simulink model "TNPC_2niveis_GridConnected"  (R2023b)
settings: Solver=FixedStepDiscrete  StartTime=0.0  StopTime=0.04  RelTol=1e-3  EnableMultiTasking=on
InitFcn:
  | %% Definition of the parameters
  | 
  | Config_TNPC_Parameters
  | 
  | %% Damping
  | 
  | Rd = 4;
  | 
  | %% PRes Gains Calculation
  | 
  | % Definicao das grandezas
  | w_cl = 1j*2*pi*800;  % Phase Crossing Frequency
  | no   = 1;           % Integral Resonant Constant
  | A    = 1;             % Carrier Amplitude
  | 
  | % Kp calculation
  | a0 = 1;
  | a1 = Rd*Cf;
  | b0 = 0;
  | b1 = Lf+Lg;
  | b2 = Rd*Lf*Cf+Rd*Lg*Cf;
  | b3 = Lf*Lg*Cf;
  | 
  | G_lcl = (a1*w_cl+a0)/(b3*w_cl^3+b2*w_cl^2+b1*w_cl+b0);
  | G_lcl = 1/(Lf*w_cl+Rf);
  | 
  | G_PWM = (1/A)*(1-w_cl*Ts/4)/(1+w_cl*Ts/4);
  | 
  | G_wc  = (Vdc/2)*K_i*G_lcl*G_PWM;
  | 
  | G_wc_abs = abs(G_wc);
  | 
  | Kp = 1/G_wc_abs;
  | 
  | % Discretized Controller Gains
  | ressonance_list = [1,5];
  | 
  | n_res = length(ressonance_list);
  | a = zeros(1,n_res);
  | b = zeros(1,n_res);
  | Ki_res = zeros(1,n_res);
  | 
  | for i = 1:n_res
  |   k = ressonance_list(i);
  |   Ki_res(i) = (2.2*Kp)/(no*T_gr);
  |   a(i) = (2*Ki_res(i)*Ts)/(4+((k*w_gr)^2)*Ts^2);
  |   b(i) = (-8+2*((k*w_gr)^2)*Ts^2)/(4+((k*w_gr)^2)*Ts^2);
  | end
undefined symbols (not defined in the file): Down, GPTRIP1SEL, K_i, K_vc, K_vdc, TZ1, Up
libraries: c2802xlib x32, c2837xDlib x3, slpidlib x2
(part 2 of 2)

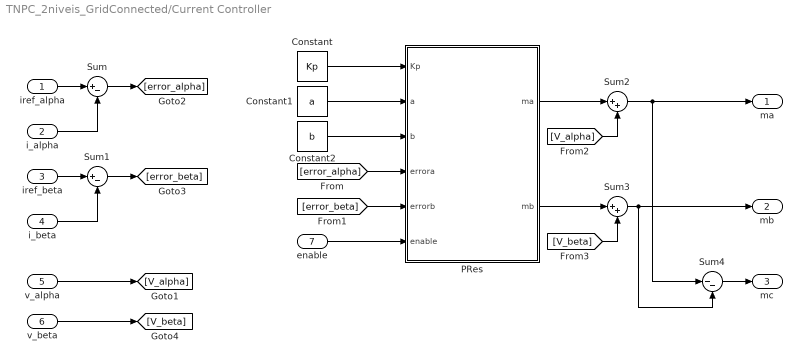
== system TNPC_2niveis_GridConnected/Current Controller ==
  iref_alpha : Inport
  i_alpha : Inport  Port=2
  iref_beta : Inport  Port=3
  i_beta : Inport  Port=4
  v_alpha : Inport  Port=5
  v_beta : Inport  Port=6
  enable : Inport  Port=7
  Constant : Constant  Value=Kp
  Constant1 : Constant  Value=a
  Constant2 : Constant  Value=b
  PRes : MATLAB Function  TreatAsAtomicUnit=on
  Sum : Sum  Inputs=|+-
  Sum1 : Sum  Inputs=|+-
  Sum2 : Sum  Inputs=|++
  Sum3 : Sum  Inputs=|++
  Sum4 : Sum  Inputs=|--
  ma : Outport
  mb : Outport  Port=2
  mc : Outport  Port=3
  wires:
  Constant/1 -> PRes/1(Kp)
  Constant1/1 -> PRes/2(a)
  Constant2/1 -> PRes/3(b)
  [error_alpha] -> PRes/4(errora)
  [error_beta] -> PRes/5(errorb)
  iref_alpha/1 -> Sum/1
  i_alpha/1 -> Sum/2
  iref_beta/1 -> Sum1/1
  i_beta/1 -> Sum1/2
  Sum1/1 -> [error_beta]
  Sum/1 -> [error_alpha]
  enable/1 -> PRes/6(enable)
  PRes/1(ma) -> Sum2/1
  Sum2/1 -> Sum4/1, ma/1
  PRes/2(mb) -> Sum3/1
  Sum3/1 -> mb/1, Sum4/2
  v_alpha/1 -> [V_alpha]
  v_beta/1 -> [V_beta]
  [V_alpha] -> Sum2/2
  [V_beta] -> Sum3/2
  Sum4/1 -> mc/1

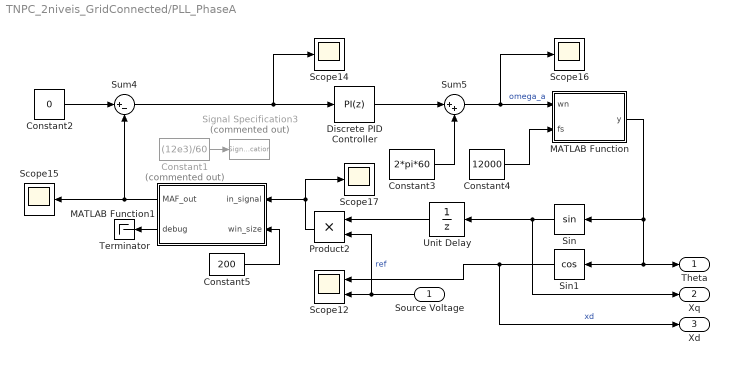
== system TNPC_2niveis_GridConnected/PLL_PhaseA ==
  Source Voltage : Inport
  Constant1 : Constant  Commented=on  Value=(12e3)/60
  Constant2 : Constant  Value=0  OutDataTypeStr=single
  Constant3 : Constant  Value=2*pi*60  OutDataTypeStr=single
  Constant4 : Constant  Value=12000  OutDataTypeStr=single
  Constant5 : Constant  Value=200  OutDataTypeStr=single
  Discrete PID Controller : slpidlib/PID Controller  Controller=PI  Form=Parallel  TimeDomain=Discrete-time  UseExternalTs=off  SampleTime=-1  IntegratorMethod=Forward Euler  FilterMethod=Forward Euler  ControllerParametersSource=internal  P=200  I=4000  UseKiTs=off  D=0  N=100  UseFilter=on  TunerSelectOption=Transfer Function Based (PID Tuner App)  InitialConditionSource=internal  InitialConditionForIntegrator=0  InitialConditionForFilter=0  DifferentiatorICPrevScaledInput=0  ExternalReset=none  TrackingMode=off  Kt=1  LimitOutput=off  SatLimitsSource=internal  UpperSaturationLimit=inf  LowerSaturationLimit=-inf  LinearizeAsGain=off  AntiWindupMode=none  Kb=1  LimitIntegrator=off  UpperIntegratorSaturationLimit=inf  LowerIntegratorSaturationLimit=-inf  POutMin=[]  POutMax=[]  IOutMin=[]  IOutMax=[]  DOutMin=[]  DOutMax=[]  NOutMin=[]  NOutMax=[]  SumOutMin=[]  SumOutMax=[]  SaturationOutMin=[]  SaturationOutMax=[]  PParamMin=[]  PParamMax=[]  IParamMin=[]  IParamMax=[]  DParamMin=[]  DParamMax=[]  NParamMin=[]  NParamMax=[]  KbParamMin=[]  KbParamMax=[]  KtParamMin=[]  KtParamMax=[]  KbOutMin=[]  KbOutMax=[]  KtOutMin=[]  KtOutMax=[]  IntegratorOutMin=[]  IntegratorOutMax=[]  FilterOutMin=[]  FilterOutMax=[]  SumI1OutMin=[]  SumI1OutMax=[]  SumI2OutMin=[]  SumI2OutMax=[]  SumI3OutMin=[]  SumI3OutMax=[]  SumI4OutMin=[]  SumI4OutMax=[]  SumDOutMin=[]  SumDOutMax=[]  DifferentiatorOutMin=[]  DifferentiatorOutMax=[]  FilterDiffOutCoefMin=[]  FilterDiffOutCoefMax=[]  ReciprocalOutMin=[]  ReciprocalOutMax=[]  SumDenOutMin=[]  SumDenOutMax=[]  SumNumOutMin=[]  SumNumOutMax=[]  DivideOutMin=[]  DivideOutMax=[]  UdiffTsProdOutMin=[]  UdiffTsProdOutMax=[]  NTsProdOutMin=[]  NTsProdOutMax=[]  UintegralTsProdOutMin=[]  UintegralTsProdOutMax=[]  UngainTsProdOutMin=[]  UngainTsProdOutMax=[]  ClampingZeroOutDataTypeStr=Inherit: Inherit via back propagation  ClampingZeroOutMin=[]  ClampingZeroOutMax=[]  FilterDenConstantOutDataTypeStr=Inherit: Inherit via back propagation  FilterDenConstantOutMin=[]  FilterDenConstantOutMax=[]  PCopyOutDataTypeStr=Inherit: Inherit via back propagation  PCopyOutMin=[]  PCopyOutMax=[]  NCopyOutDataTypeStr=Inherit: Inherit via back propagation  NCopyOutMin=[]  NCopyOutMax=[]  IntegratorContinuousStateAttributes=''  IntegratorStateMustResolveToSignalObject=off  IntegratorRTWStateStorageClass=Auto  FilterContinuousStateAttributes=''  FilterStateMustResolveToSignalObject=off  FilterRTWStateStorageClass=Auto  ParallelPVariant=InternalParameters  IdealPVariant=Disabled  IVariant=InternalParameters  DVariant=Disabled  IntegratorVariant=Discrete  SatVariant=Disabled  AWVariant=Passthrough  PCopyVariant=Disabled  TRVariant=Disabled  FdbkBlocksVariant=Forward  IdealPFdbkVariant=Disabled  SatFdbkVariant=Disabled  DerivativeFilterVariant=Disabled  NVariant=Disabled  NCopyVariant=Disabled_SignalSpec  FilterICVariant=Disabled  IntegratorICVariant=InternalICs  ExternalResetVariant=Disabled  TRSumVariant=Passthrough  SumFdbkVariant=Disabled  SumVariant=Sum_PI  TsampFilterVariant=InternalTs  TsampNgainVariant=Passthrough  TsampIntegralVariant=Disabled_SignalSpec  ExternalSaturationOutDataTypeStr=Inherit: Same as second input
  MATLAB Function : MATLAB Function  TreatAsAtomicUnit=on
  MATLAB Function1 : MATLAB Function  TreatAsAtomicUnit=on
  Product2 : Product
  Scope12 : Scope  NumInputPorts=2
  Scope{14..17} (4 alike) : Scope
  Signal Specification3 : SignalSpecification  Commented=on  Dimensions=[1 1]
  Sin : Trigonometry
  Sin1 : Trigonometry  Operator=cos
  Sum4 : Sum  Inputs=|+-
  Sum5 : Sum  Inputs=|++
  Terminator : Terminator
  Unit Delay : UnitDelay  SampleTime=-1  HasFrameUpgradeWarning=on
  Theta : Outport
  Xq : Outport  Port=2
  Xd : Outport  Port=3
  wires:
  Constant1/1 -> Signal Specification3/1
  Constant4/1 -> MATLAB Function/2(fs)
  Sum5/1 -> MATLAB Function/1(wn), Scope16/1  "omega_a"
  Source Voltage/1 -> Scope12/2, Product2/2  "ref"
  Constant3/1 -> Sum5/2
  Unit Delay/1 -> Product2/1
  Constant2/1 -> Sum4/1
  Sum4/1 -> Scope14/1, Discrete PID Controller/1
  Sin/1 -> Unit Delay/1, Xq/1
  Sin1/1 -> Scope12/1, Xd/1  "xd"
  Product2/1 -> MATLAB Function1/1(in_signal), Scope17/1
  MATLAB Function/1(y) -> Sin/1, Sin1/1, Theta/1
  Discrete PID Controller/1 -> Sum5/1
  MATLAB Function1/1(MAF_out) -> Sum4/2, Scope15/1
  Constant5/1 -> MATLAB Function1/2(win_size)
  MATLAB Function1/2(debug) -> Terminator/1

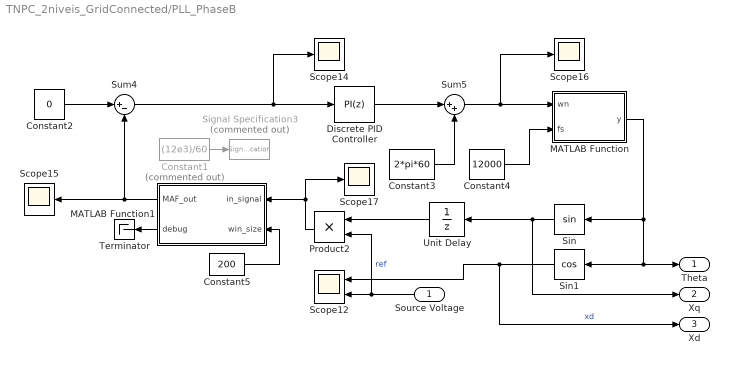
== system TNPC_2niveis_GridConnected/PLL_PhaseB ==
  Source Voltage : Inport
  Constant1 : Constant  Commented=on  Value=(12e3)/60
  Constant2 : Constant  Value=0  OutDataTypeStr=single
  Constant3 : Constant  Value=2*pi*60  OutDataTypeStr=single
  Constant4 : Constant  Value=12000  OutDataTypeStr=single
  Constant5 : Constant  Value=200  OutDataTypeStr=single
  Discrete PID Controller : slpidlib/PID Controller  Controller=PI  Form=Parallel  TimeDomain=Discrete-time  UseExternalTs=off  SampleTime=-1  IntegratorMethod=Forward Euler  FilterMethod=Forward Euler  ControllerParametersSource=internal  P=200  I=4000  UseKiTs=off  D=0  N=100  UseFilter=on  TunerSelectOption=Transfer Function Based (PID Tuner App)  InitialConditionSource=internal  InitialConditionForIntegrator=0  InitialConditionForFilter=0  DifferentiatorICPrevScaledInput=0  ExternalReset=none  TrackingMode=off  Kt=1  LimitOutput=off  SatLimitsSource=internal  UpperSaturationLimit=inf  LowerSaturationLimit=-inf  LinearizeAsGain=off  AntiWindupMode=none  Kb=1  LimitIntegrator=off  UpperIntegratorSaturationLimit=inf  LowerIntegratorSaturationLimit=-inf  POutMin=[]  POutMax=[]  IOutMin=[]  IOutMax=[]  DOutMin=[]  DOutMax=[]  NOutMin=[]  NOutMax=[]  SumOutMin=[]  SumOutMax=[]  SaturationOutMin=[]  SaturationOutMax=[]  PParamMin=[]  PParamMax=[]  IParamMin=[]  IParamMax=[]  DParamMin=[]  DParamMax=[]  NParamMin=[]  NParamMax=[]  KbParamMin=[]  KbParamMax=[]  KtParamMin=[]  KtParamMax=[]  KbOutMin=[]  KbOutMax=[]  KtOutMin=[]  KtOutMax=[]  IntegratorOutMin=[]  IntegratorOutMax=[]  FilterOutMin=[]  FilterOutMax=[]  SumI1OutMin=[]  SumI1OutMax=[]  SumI2OutMin=[]  SumI2OutMax=[]  SumI3OutMin=[]  SumI3OutMax=[]  SumI4OutMin=[]  SumI4OutMax=[]  SumDOutMin=[]  SumDOutMax=[]  DifferentiatorOutMin=[]  DifferentiatorOutMax=[]  FilterDiffOutCoefMin=[]  FilterDiffOutCoefMax=[]  ReciprocalOutMin=[]  ReciprocalOutMax=[]  SumDenOutMin=[]  SumDenOutMax=[]  SumNumOutMin=[]  SumNumOutMax=[]  DivideOutMin=[]  DivideOutMax=[]  UdiffTsProdOutMin=[]  UdiffTsProdOutMax=[]  NTsProdOutMin=[]  NTsProdOutMax=[]  UintegralTsProdOutMin=[]  UintegralTsProdOutMax=[]  UngainTsProdOutMin=[]  UngainTsProdOutMax=[]  ClampingZeroOutDataTypeStr=Inherit: Inherit via back propagation  ClampingZeroOutMin=[]  ClampingZeroOutMax=[]  FilterDenConstantOutDataTypeStr=Inherit: Inherit via back propagation  FilterDenConstantOutMin=[]  FilterDenConstantOutMax=[]  PCopyOutDataTypeStr=Inherit: Inherit via back propagation  PCopyOutMin=[]  PCopyOutMax=[]  NCopyOutDataTypeStr=Inherit: Inherit via back propagation  NCopyOutMin=[]  NCopyOutMax=[]  IntegratorContinuousStateAttributes=''  IntegratorStateMustResolveToSignalObject=off  IntegratorRTWStateStorageClass=Auto  FilterContinuousStateAttributes=''  FilterStateMustResolveToSignalObject=off  FilterRTWStateStorageClass=Auto  ParallelPVariant=InternalParameters  IdealPVariant=Disabled  IVariant=InternalParameters  DVariant=Disabled  IntegratorVariant=Discrete  SatVariant=Disabled  AWVariant=Passthrough  PCopyVariant=Disabled  TRVariant=Disabled  FdbkBlocksVariant=Forward  IdealPFdbkVariant=Disabled  SatFdbkVariant=Disabled  DerivativeFilterVariant=Disabled  NVariant=Disabled  NCopyVariant=Disabled_SignalSpec  FilterICVariant=Disabled  IntegratorICVariant=InternalICs  ExternalResetVariant=Disabled  TRSumVariant=Passthrough  SumFdbkVariant=Disabled  SumVariant=Sum_PI  TsampFilterVariant=InternalTs  TsampNgainVariant=Passthrough  TsampIntegralVariant=Disabled_SignalSpec  ExternalSaturationOutDataTypeStr=Inherit: Same as second input
  MATLAB Function : MATLAB Function  TreatAsAtomicUnit=on
  MATLAB Function1 : MATLAB Function  TreatAsAtomicUnit=on
  Product2 : Product
  Scope12 : Scope  NumInputPorts=2
  Scope{14..17} (4 alike) : Scope
  Signal Specification3 : SignalSpecification  Commented=on  Dimensions=[1 1]
  Sin : Trigonometry
  Sin1 : Trigonometry  Operator=cos
  Sum4 : Sum  Inputs=|+-
  Sum5 : Sum  Inputs=|++
  Terminator : Terminator
  Unit Delay : UnitDelay  SampleTime=-1  HasFrameUpgradeWarning=on
  Theta : Outport
  Xq : Outport  Port=2
  Xd : Outport  Port=3
  wires:
  MATLAB Function1/2(debug) -> Terminator/1
  Constant5/1 -> MATLAB Function1/2(win_size)
  MATLAB Function1/1(MAF_out) -> Scope15/1, Sum4/2
  Discrete PID Controller/1 -> Sum5/1
  MATLAB Function/1(y) -> Theta/1, Sin1/1, Sin/1
  Product2/1 -> MATLAB Function1/1(in_signal), Scope17/1
  Sin1/1 -> Xd/1, Scope12/1  "xd"
  Sin/1 -> Xq/1, Unit Delay/1
  Sum4/1 -> Discrete PID Controller/1, Scope14/1
  Constant2/1 -> Sum4/1
  Unit Delay/1 -> Product2/1
  Constant3/1 -> Sum5/2
  Source Voltage/1 -> Product2/2, Scope12/2  "ref"
  Sum5/1 -> Scope16/1, MATLAB Function/1(wn)
  Constant4/1 -> MATLAB Function/2(fs)
  Constant1/1 -> Signal Specification3/1

== matlab function TNPC_2niveis_GridConnected/MATLAB Function11 ==
  data: i_rms input; error_overcurrent output; error_ac_overvoltage output; error_dc_overvoltage output; error_unbalance output; error_low_Vdc output; enable_contactor_out output; enable_PreCharge_out output; enable_PWM_out output; I_limit input; V_rms input; V_limit input; V_dc input; Vdc_limit input; V_unb input; Vunb_limit input; enable_relay input; enable_PWM input; enable_PreCharge input; error_reset input; error_reset_out output; out_gpio output
function [error_overcurrent, error_ac_overvoltage, error_dc_overvoltage, error_unbalance, error_low_Vdc, enable_contactor_out, enable_PreCharge_out, enable_PWM_out, error_reset_out, out_gpio] = TNPC_Protection(i_rms, I_limit, V_rms, V_limit, V_dc, Vdc_limit, V_unb, Vunb_limit, enable_relay, enable_PWM, enable_PreCharge, error_reset)

% Persistent variables definition
persistent error_flag
persistent error_overcurrent_p
persistent error_ac_overvoltage_p
persistent error_dc_overvoltage_p
persistent error_unbalance_p
persistent error_low_Vdc_p
if isempty(error_flag)
    error_flag = single(0);
    error_overcurrent_p    = single(0);
    error_ac_overvoltage_p = single(0);
    error_dc_overvoltage_p = single(0);
    error_unbalance_p      = single(0);
    error_low_Vdc_p        = single(0);
end

% Check for errors
if max(i_rms) > I_limit
    error_overcurrent = single(1);
    error_overcurrent_p = single(1);
else
    error_overcurrent = single(0);
end

if V_dc > Vdc_limit
    error_dc_overvoltage = single(1);
    error_dc_overvoltage_p = single(1);
else
    error_dc_overvoltage = single(0);  
end

if V_unb > Vunb_limit
    error_unbalance = single(1);
    error_unbalance_p = single(1);
else
    error_unbalance = single(0);
end

if max(V_rms) > V_limit
    error_ac_overvoltage = single(1);
    error_ac_overvoltage_p = single(1);
else
    error_ac_overvoltage = single(0);  
end

if V_dc*500 < sqrt(2)*max(V_rms)*250
    error_low_Vdc = single(1);
    error_low_Vdc_p = single(1);
else
    error_low_Vdc = single(0);
end

% Raise the error flag
if (error_overcurrent == 1) || (error_dc_overvoltage == 1) || (error_unbalance == 1) || (error_ac_overvoltage == 1) || (error_low_Vdc == 1)
    error_flag = single(1);
end

% Reset logic
if error_flag == 1 && error_reset == 1 && error_overcurrent == 0 && error_dc_overvoltage == 0 && error_ac_overvoltage == 0 && error_unbalance == 0 && error_low_Vdc == 0
    % Clear the persistent variables
    error_flag = single(0);
    error_overcurrent_p    = single(0);
    error_ac_overvoltage_p = single(0);
    error_dc_overvoltage_p = single(0);
    error_unbalance_p      = single(0);
    error_low_Vdc_p        = single(0);
    % Send 0 to the reset signal
    error_reset_out = single(0);
else
    error_reset_out = error_reset;
end

% Enable signals output
if error_flag == 1
    enable_contactor_out = single(0);
    enable_PWM_out   = single(0);
    enable_PreCharge_out = single(0);
else
    enable_contactor_out = enable_relay;
    enable_PWM_out   = enable_PWM;
    enable_PreCharge_out = enable_PreCharge;
end

if (error_overcurrent_p == 1) || (error_dc_overvoltage_p == 1) || (error_unbalance_p == 1) || (error_ac_overvoltage_p == 1) || (error_low_Vdc_p == 1)
    out_gpio = single(1);
else
    out_gpio = single(0);
end

== matlab function TNPC_2niveis_GridConnected/Current Controller/PRes ==
  data: Kp input; a input; b input; errora input; ma output; errorb input; mb output; enable input
function [ma, mb] = PResCurrent(Kp, a, b, errora, errorb, enable)

%Controller modeled in abc frame, considering p.u. values

%%% Variables Definition
%%%%#########################################################
%%%%######################################################### 

nRes = length(a);

max_pu = single(1.0);

%Proportional part variable
%Phase a
persistent pia
    if isempty(pia)
        pia = single(0.0);
    end
%Phase b    
persistent pib
    if isempty(pib)
        pib = single(0.0);
    end 
    
%Resonant parts variables
%Phase a
persistent presa
    if isempty(presa)
        presa = zeros(1,nRes);
    end
persistent presa_1d %1 sample delay
    if isempty(presa_1d)
        presa_1d = zeros(1,nRes);
    end    
persistent presa_2d %2 samples delay
    if isempty(presa_2d)
        presa_2d = zeros(1,nRes);
    end
persistent presOUT_ia
    if isempty(presOUT_ia)
        presOUT_ia = single(0.0);
    end
    
%Phase b
persistent presb
    if isempty(presb)
        presb = zeros(1,nRes);
    end
persistent presb_1d %1 sample delay
    if isempty(presb_1d)
        presb_1d = zeros(1,nRes);
    end    
persistent presb_2d %2 samples delay
    if isempty(presb_2d)
        presb_2d = zeros(1,nRes);
    end
persistent presOUT_ib
    if isempty(presOUT_ib)
        presOUT_ib = single(0.0);
    end

%Error variables
%Phase a
% persistent errora %Actual error
%     if isempty(errora)
%         errora = 0.0;
%     end
persistent errora_0d %Actual error to delay
    if isempty(errora_0d)
        errora_0d = single(0.0);
    end
persistent errora_1d %1 sample delay
    if isempty(errora_1d)
        errora_1d = single(0.0);
    end    
persistent errora_2d %2 sample delay
    if isempty(errora_2d)
        errora_2d = single(0.0);
    end   
%Phase b
% persistent errorb %Actual error
%     if isempty(errorb)
%         errorb = 0.0;
%     end
persistent errorb_0d %Actual error to delay
    if isempty(errorb_0d)
        errorb_0d = single(0.0);
    end
persistent errorb_1d %1 sample delay
    if isempty(errorb_1d)
        errorb_1d = single(0.0);
    end    
persistent errorb_2d %2 sample delay
    if isempty(errorb_2d)
        errorb_2d = single(0.0);
    end

%%% Enable logic
%%%%#########################################################
%%%%#########################################################

if ~enable 
    % Define safe outputs
    ma = single(0.0);
    mb = single(0.0);
    mc = single(0.0);
    
    % Reset history registers for bumpless transfer
    pia = single(0.0); pib = single(0.0);
    
    presa       = zeros(1,nRes);
    presa_1d    = zeros(1,nRes);
    presa_2d    = zeros(1,nRes);
    presOUT_ia  = single(0.0);
    
    presb       = zeros(1,nRes);
    presb_1d    = zeros(1,nRes);
    presb_2d    = zeros(1,nRes);
    presOUT_ib  = single(0.0);
    
    errora_0d = single(0.0); errora_1d = single(0.0); errora_2d = single(0.0);
    errorb_0d = single(0.0); errorb_1d = single(0.0); errorb_2d = single(0.0);
    
    % Exit the function completely
    return; 
end

%%% PRes Current Controllers
%%%%#########################################################
%%%%#########################################################

%Proportional part
pia = errora*Kp;
pib = errorb*Kp;
    
    %Saturation - a
    if pia > max_pu 
        pia = max_pu;
    end
    if pia < -1*max_pu
        pia = -1*max_pu;
    end
    %Saturation - b
    if pib > max_pu
        pib = max_pu;
    end
    if pib < -1*max_pu
        pib = -1*max_pu;
    end   
    
    % %Anti-windup - a
    % if pia > 0.0
    %     limit_ia = max_pu - pia;
    % else
    %     limit_ia = 1 + pia;
    % end
    %  %Anti-windup - b
    % if pib > 0.0
    %     limit_ib = max_pu - pib;
    % else
    %     limit_ib = 1 + pib;
    % end
%     %Anti-windup - c
%     if pic > 0.0
%         limit_ic = max_pu - pic;
%     else
%         limit_ic = 1 + pic;
%     end    
    
    
%Resonant part
errora_2d = errora_1d;
errora_1d = errora_0d;
errora_0d = errora;

errorb_2d = errorb_1d;
errorb_1d = errorb_0d;
errorb_0d = errorb;
        
for i=1:nRes

    %leg a
    presa_2d(i) = presa_1d(i);
	presa_1d(i) = presa(i);
	presa(i) = a(i)*errora -a(i)*errora_2d - b(i)*presa_1d(i) - presa_2d(i);    
    % if presa(i) > limit_ia
    %     presa(i) = limit_ia;
    % end
    % if presa(i) < -1*limit_ia
    %     presa(i) = -1*limit_ia;
    % end
 
    %leg b
    presb_2d(i) = presb_1d(i);
	presb_1d(i) = presb(i);
	presb(i) = a(i)*errorb -a(i)*errorb_2d - b(i)*presb_1d(i) - presb_2d(i);    
    % if presb(i) > limit_ib
    %     presb(i) = limit_ib;
    % end
    % if presb(i) < -1*limit_ib
    %     presb(i) = -1*limit_ib;
    % end  
    
end

presOUT_ia = pia;
presOUT_ib = pib;

for i=1:nRes
    presOUT_ia = presOUT_ia + presa(i);
    presOUT_ib = presOUT_ib + presb(i);  
end

%Output for PWM
ma = presOUT_ia;
        %Saturation - ta
        if ma > max_pu 
            ma = max_pu;
        end
        if ma < -1*max_pu
            ma = -1*max_pu;
        end

mb = presOUT_ib;
        %Saturation - tb
        if mb > max_pu 
            mb = max_pu;
        end
        if mb < -1*max_pu
            mb = -1*max_pu;
        end
        
end

== matlab function TNPC_2niveis_GridConnected/PLL_PhaseB/MATLAB Function ==
  data: wn input; y output; fs input
function y = Int_Sat(wn,fs)

persistent theta_n;
    if isempty(theta_n)
         theta_n = single(0.00);
    end
    
    theta_n = theta_n + wn*(1/fs);
    
    if theta_n >= 2*pi
        theta_n = theta_n - 2*pi;
    end
y = theta_n;

== matlab function TNPC_2niveis_GridConnected/PLL_PhaseA/MATLAB Function ==
  data: wn input; y output; fs input
function y = Int_Sat(wn,fs)

persistent theta_n;
    if isempty(theta_n)
         theta_n = single(0.00);
    end
    
    theta_n = theta_n + wn*(1/fs);
    
    if theta_n >= 2*pi
        theta_n = theta_n - 2*pi;
    end
y = theta_n;

== matlab function TNPC_2niveis_GridConnected/PLL_PhaseA/MATLAB Function1 ==
  data: MAF_out output; in_signal input; debug output; win_size input

function [MAF_out, debug] = MAF(in_signal,win_size)

% persistent win_size;
%     if isempty(win_size)
%         win_size = 200;
%     end

%win_size: window size (number of points in one fundamental cycle)
%Sampling frequency (fs) -> Sampling time (Ts = 1/ fs)

% persistent win_size;
%     if isempty(win_size)
%         win_size = window_size;
%     end
% persistent in_signal;
%     if isempty(in_signal)
%         in_signal = input_signal;
%     end    
persistent buffer;
    if isempty(buffer)
        %buffer = zeros(1,win_size);
        buffer = zeros(1,200); 
    end
persistent sum_buffer;
    if isempty(sum_buffer)
        sum_buffer = single(0.0);
    end
persistent array_pos;
    if isempty(array_pos)
        array_pos = 1;
    end
persistent MAF;
    if isempty(MAF)
        MAF = single(0.0);
    end


%%%%%%%%%%%%%%%%%%%%%%%%%%%
%Moving Average Filter (MAF)

%Reset buffer if window size is extrapolated
if array_pos == (win_size + 1)

    array_pos = 1; %Reset

end

    %MAF update and summing
    sum_buffer = sum_buffer + in_signal - buffer(1,array_pos);
    buffer(1,array_pos) = in_signal;
    
    %MAF Output
    MAF = sum_buffer/win_size;

%Going for the next position
array_pos = array_pos + 1;

MAF_out = MAF; %MAF output

debug = 10;

== matlab function TNPC_2niveis_GridConnected/PLL_PhaseB/MATLAB Function1 ==
  data: MAF_out output; in_signal input; debug output; win_size input

function [MAF_out, debug] = MAF(in_signal,win_size)

% persistent win_size;
%     if isempty(win_size)
%         win_size = 200;
%     end

%win_size: window size (number of points in one fundamental cycle)
%Sampling frequency (fs) -> Sampling time (Ts = 1/ fs)

% persistent win_size;
%     if isempty(win_size)
%         win_size = window_size;
%     end
% persistent in_signal;
%     if isempty(in_signal)
%         in_signal = input_signal;
%     end    
persistent buffer;
    if isempty(buffer)
        %buffer = zeros(1,win_size);
        buffer = zeros(1,200); 
    end
persistent sum_buffer;
    if isempty(sum_buffer)
        sum_buffer = single(0.0);
    end
persistent array_pos;
    if isempty(array_pos)
        array_pos = 1;
    end
persistent MAF;
    if isempty(MAF)
        MAF = single(0.0);
    end


%%%%%%%%%%%%%%%%%%%%%%%%%%%
%Moving Average Filter (MAF)

%Reset buffer if window size is extrapolated
if array_pos == (win_size + 1)

    array_pos = 1; %Reset

end

    %MAF update and summing
    sum_buffer = sum_buffer + in_signal - buffer(1,array_pos);
    buffer(1,array_pos) = in_signal;
    
    %MAF Output
    MAF = sum_buffer/win_size;

%Going for the next position
array_pos = array_pos + 1;

MAF_out = MAF; %MAF output

debug = 10;

== matlab function TNPC_2niveis_GridConnected/RMS_fcn ==
  data: RMSin input; yout output
function yout = fcn(RMSin)

win = 200;

persistent sampleRMS
    if isempty(sampleRMS)
        sampleRMS = single(0.0);
    end
    if sampleRMS>=win
        sampleRMS = single(0.0);
    end

persistent RMSout
if isempty(RMSout)
    RMSout = single(0.0);
end    
persistent sumRMS
if isempty(sumRMS)
    sumRMS = single(0.0);
end
persistent RMSinArray
     if isempty(RMSinArray)
         RMSinArray = zeros(1,win);
     end

sampleRMS = sampleRMS + 1;      

%RMS of Input Signal
sumRMS = sumRMS + RMSin*RMSin - RMSinArray(1,sampleRMS);
RMSinArray(1,sampleRMS) = RMSin*RMSin;
if sumRMS>=0.0
    RMSout = sqrt(sumRMS/win);
end

%RMSout = RMSout_temp;

yout = RMSout;

== matlab function TNPC_2niveis_GridConnected/RMS_fcn1 ==
  data: RMSin input; yout output
function yout = fcn(RMSin)

win = 200;

persistent sampleRMS
    if isempty(sampleRMS)
        sampleRMS = single(0.0);
    end
    if sampleRMS>=win
        sampleRMS = single(0.0);
    end

persistent RMSout
if isempty(RMSout)
    RMSout = single(0.0);
end    
persistent sumRMS
if isempty(sumRMS)
    sumRMS = single(0.0);
end
persistent RMSinArray
     if isempty(RMSinArray)
         RMSinArray = zeros(1,win);
     end

sampleRMS = sampleRMS + 1;      

%RMS of Input Signal
sumRMS = sumRMS + RMSin*RMSin - RMSinArray(1,sampleRMS);
RMSinArray(1,sampleRMS) = RMSin*RMSin;
if sumRMS>=0.0
    RMSout = sqrt(sumRMS/win);
end

%RMSout = RMSout_temp;

yout = RMSout;

== matlab function TNPC_2niveis_GridConnected/RMS_fcn2 ==
  data: RMSin input; yout output
function yout = fcn(RMSin)

win = 200;

persistent sampleRMS
    if isempty(sampleRMS)
        sampleRMS = single(0.0);
    end
    if sampleRMS>=win
        sampleRMS = single(0.0);
    end

persistent RMSout
if isempty(RMSout)
    RMSout = single(0.0);
end    
persistent sumRMS
if isempty(sumRMS)
    sumRMS = single(0.0);
end
persistent RMSinArray
     if isempty(RMSinArray)
         RMSinArray = zeros(1,win);
     end

sampleRMS = sampleRMS + 1;      

%RMS of Input Signal
sumRMS = sumRMS + RMSin*RMSin - RMSinArray(1,sampleRMS);
RMSinArray(1,sampleRMS) = RMSin*RMSin;
if sumRMS>=0.0
    RMSout = sqrt(sumRMS/win);
end

%RMSout = RMSout_temp;

yout = RMSout;

== matlab function TNPC_2niveis_GridConnected/RMS_fcn3 ==
  data: RMSin input; yout output
function yout = fcn(RMSin)

win = 200;

persistent sampleRMS
    if isempty(sampleRMS)
        sampleRMS = single(0.0);
    end
    if sampleRMS>=win
        sampleRMS = single(0.0);
    end

persistent RMSout
if isempty(RMSout)
    RMSout = single(0.0);
end    
persistent sumRMS
if isempty(sumRMS)
    sumRMS = single(0.0);
end
persistent RMSinArray
     if isempty(RMSinArray)
         RMSinArray = zeros(1,win);
     end

sampleRMS = sampleRMS + 1;      

%RMS of Input Signal
sumRMS = sumRMS + RMSin*RMSin - RMSinArray(1,sampleRMS);
RMSinArray(1,sampleRMS) = RMSin*RMSin;
if sumRMS>=0.0
    RMSout = sqrt(sumRMS/win);
end

%RMSout = RMSout_temp;

yout = RMSout;

== matlab function TNPC_2niveis_GridConnected/RMS_fcn4 ==
  data: RMSin input; yout output
function yout = fcn(RMSin)

win = 200;

persistent sampleRMS
    if isempty(sampleRMS)
        sampleRMS = single(0.0);
    end
    if sampleRMS>=win
        sampleRMS = single(0.0);
    end

persistent RMSout
if isempty(RMSout)
    RMSout = single(0.0);
end    
persistent sumRMS
if isempty(sumRMS)
    sumRMS = single(0.0);
end
persistent RMSinArray
     if isempty(RMSinArray)
         RMSinArray = zeros(1,win);
     end

sampleRMS = sampleRMS + 1;      

%RMS of Input Signal
sumRMS = sumRMS + RMSin*RMSin - RMSinArray(1,sampleRMS);
RMSinArray(1,sampleRMS) = RMSin*RMSin;
if sumRMS>=0.0
    RMSout = sqrt(sumRMS/win);
end

%RMSout = RMSout_temp;

yout = RMSout;

== matlab function TNPC_2niveis_GridConnected/RMS_fcn5 ==
  data: RMSin input; yout output
function yout = fcn(RMSin)

win = 200;

persistent sampleRMS
    if isempty(sampleRMS)
        sampleRMS = single(0.0);
    end
    if sampleRMS>=win
        sampleRMS = single(0.0);
    end

persistent RMSout
if isempty(RMSout)
    RMSout = single(0.0);
end    
persistent sumRMS
if isempty(sumRMS)
    sumRMS = single(0.0);
end
persistent RMSinArray
     if isempty(RMSinArray)
         RMSinArray = zeros(1,win);
     end

sampleRMS = sampleRMS + 1;      

%RMS of Input Signal
sumRMS = sumRMS + RMSin*RMSin - RMSinArray(1,sampleRMS);
RMSinArray(1,sampleRMS) = RMSin*RMSin;
if sumRMS>=0.0
    RMSout = sqrt(sumRMS/win);
end

%RMSout = RMSout_temp;

yout = RMSout;
